simulink model "chapter3_twoareafrequencycontrol_linearmodel"  (R2013b)
settings: Solver=ode45  StartTime=0.0  StopTime=600  MaxStep=0.01  RelTol=1e-3
InitFcn:
  | R1 = 0.05;
  | R2 = 0.1;
  | H = 5;
  | D1 =1;
  | T =1;
settings Model: Creator=linglingfan  LastModifiedBy=linglingfan

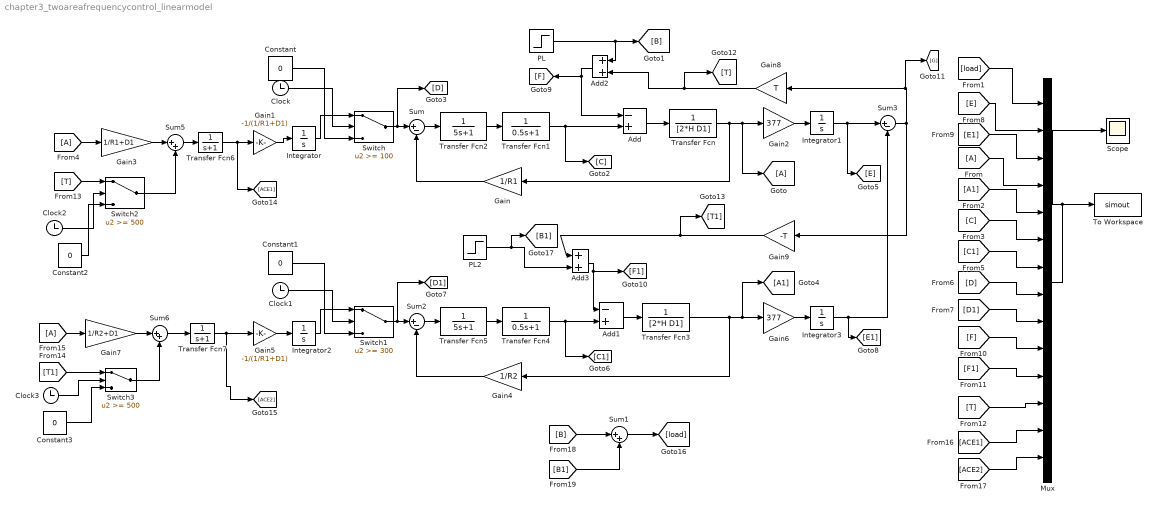
== system chapter3_twoareafrequencycontrol_linearmodel ==
  Add : Sum  Inputs=-+
  Add1 : Sum  Inputs=-+
  Add2 : Sum
  Add3 : Sum
  Clock{,1..3} (4 alike) : Clock
  Constant{,1..3} (4 alike) : Constant  Value=0
  Gain : Gain  Gain=1/R1
  Gain1 : Gain  Gain=-1/(1/R1+D1)
  Gain2 : Gain  Gain=377
  Gain3 : Gain  Gain=1/R1+D1
  Gain4 : Gain  Gain=1/R2
  Gain5 : Gain  Gain=-1/(1/R1+D1)
  Gain6 : Gain  Gain=377
  Gain7 : Gain  Gain=1/R2+D1
  Gain8 : Gain  Gain=T
  Gain9 : Gain  Gain=-T
  Integrator{,1..3} (4 alike) : Integrator
  Mux : Mux  Inputs=14
  PL : Step  Time=10  After=0.2  SampleTime=0
  PL2 : Step  Time=210  After=0.3  SampleTime=0
  Scope : Scope
  Sum : Sum  Inputs=|+-
  Sum1 : Sum  Inputs=|++
  Sum2 : Sum  Inputs=|+-
  Sum3 : Sum  Inputs=|+-
  Sum5 : Sum  Inputs=|++
  Sum6 : Sum  Inputs=|++
  Switch : Switch  Threshold=100
  Switch1 : Switch  Threshold=300
  Switch2 : Switch  Threshold=500
  Switch3 : Switch  Threshold=500
  To Workspace : ToWorkspace  VariableName=simout  SampleTime=-1  SaveFormat=Timeseries
  Transfer Fcn : TransferFcn  Denominator=[2*H D1]
  Transfer Fcn1 : TransferFcn  Denominator=[0.5 1]
  Transfer Fcn2 : TransferFcn  Denominator=[5 1]
  Transfer Fcn3 : TransferFcn  Denominator=[2*H D1]
  Transfer Fcn4 : TransferFcn  Denominator=[0.5 1]
  Transfer Fcn5 : TransferFcn  Denominator=[5 1]
  Transfer Fcn6 : TransferFcn  Denominator=[1 1]
  Transfer Fcn7 : TransferFcn  Denominator=[1 1]
  wires:
  Add/1 -> Transfer Fcn/1
  Transfer Fcn1/1 -> Add/2, [C]
  Transfer Fcn/1 -> [A], Gain2/1, Gain/1
  Gain1/1 -> Integrator/1
  Mux/1 -> Scope/1, To Workspace/1
  Sum/1 -> Transfer Fcn2/1
  Transfer Fcn2/1 -> Transfer Fcn1/1
  Switch/1 -> [D], Sum/1
  Clock/1 -> Switch/2
  Constant/1 -> Switch/3
  Integrator/1 -> Switch/1
  Gain/1 -> Sum/2
  Gain2/1 -> Integrator1/1
  Add1/1 -> Transfer Fcn3/1
  Transfer Fcn4/1 -> [C1], Add1/2
  Transfer Fcn3/1 -> [A1], Gain6/1, Gain4/1
  Gain5/1 -> Integrator2/1
  Sum2/1 -> Transfer Fcn5/1
  Transfer Fcn5/1 -> Transfer Fcn4/1
  Switch1/1 -> [D1], Sum2/1
  Clock1/1 -> Switch1/2
  Constant1/1 -> Switch1/3
  Integrator2/1 -> Switch1/1
  Gain4/1 -> Sum2/2
  Gain6/1 -> Integrator3/1
  Integrator1/1 -> [E], Sum3/1
  Integrator3/1 -> [E1], Sum3/2
  Sum3/1 -> Gain9/1, [G], Gain8/1
  Gain8/1 -> [T], Add2/2
  [load] -> Mux/1
  [C] -> Mux/6
  [C1] -> Mux/7
  [A1] -> Mux/5
  [D] -> Mux/8
  [A] -> Mux/4
  [E1] -> Mux/3
  [D1] -> Mux/9
  [E] -> Mux/2
  PL/1 -> Add2/1, [B]
  Add2/1 -> Add/1, [F]
  PL2/1 -> [B1], Add3/2
  Add3/1 -> [F1], Add1/1
  Gain9/1 -> [T1], Add3/1
  [F] -> Mux/10
  [F1] -> Mux/11
  [T] -> Mux/12
  [A] -> Gain3/1
  Gain3/1 -> Sum5/1
  [A] -> Gain7/1
  Gain7/1 -> Sum6/1
  [ACE1] -> Mux/13
  [ACE2] -> Mux/14
  Sum1/1 -> [load]
  [B] -> Sum1/1
  [B1] -> Sum1/2
  Sum5/1 -> Transfer Fcn6/1
  [T] -> Switch2/1
  Switch2/1 -> Sum5/2
  Clock2/1 -> Switch2/2
  Constant2/1 -> Switch2/3
  Switch3/1 -> Sum6/2
  [T1] -> Switch3/1
  Constant3/1 -> Switch3/3
  Clock3/1 -> Switch3/2
  Sum6/1 -> Transfer Fcn7/1
  Transfer Fcn6/1 -> [ACE1], Gain1/1
  Transfer Fcn7/1 -> [ACE2], Gain5/1
